simulink model "Ex3"  (R2020a)
settings: Solver=ode45  StartTime=0.0  StopTime=120  RelTol=1e-3
model workspace (MAT data in the model file):
  Ki = 40
  Kp = 800
  b = 50
  m = 1000
  u = 500
settings Model: DataDictionary=CruiseControldata.sldd  Creator=aishw  LastModifiedBy=aishw
settings DebuggingCC: AlgebraicLoopMsg=none

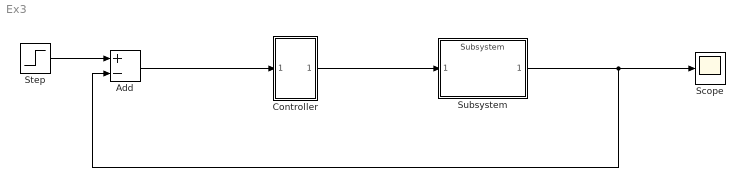
== system Ex3 ==
  Add : Sum  Inputs=+-
  Controller : Subsystem
      mask Display: disp('PI')
  Scope : Scope
  Step : Step  Time=0  After=u  SampleTime=0
  Subsystem : ModelReference  ModelNameDialog=Subsystem  ModelReferenceVersion=1.7
  wires:
  Subsystem/1 -> Scope/1, Add/2
  Step/1 -> Add/1
  Add/1 -> Controller/1(In1)
  Controller/1(Out1) -> Subsystem/1

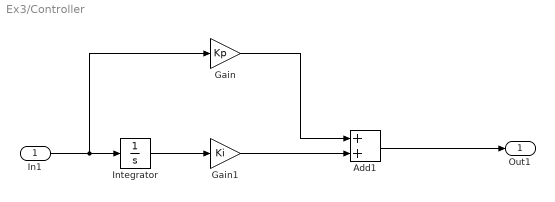
== system Ex3/Controller ==
  In1 : Inport
  Add1 : Sum
  Gain : Gain  Gain=Kp
  Gain1 : Gain  Gain=Ki
  Integrator : Integrator
  Out1 : Outport
  wires:
  In1/1 -> Gain/1, Integrator/1
  Gain1/1 -> Add1/2
  Gain/1 -> Add1/1
  Integrator/1 -> Gain1/1
  Add1/1 -> Out1/1
